simulink model "lab_modulation_am"  (R2022a)
settings: Solver=VariableStepAuto  StartTime=0.0  StopTime=10.0  RelTol=1e-3
libraries: dspfdesign x1
settings Model: Creator=salgi  LastModifiedBy=salgi

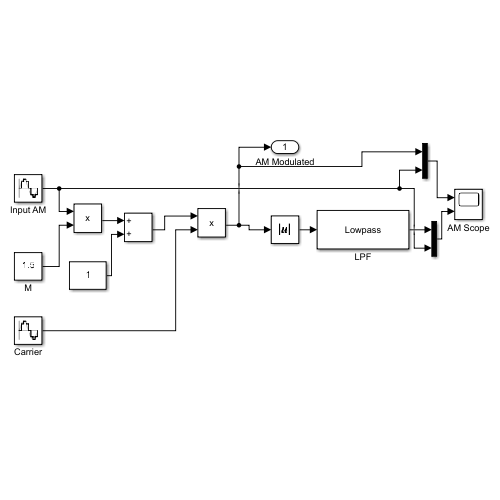
[thumbnail: Simulink's stored preview of the top-level diagram]
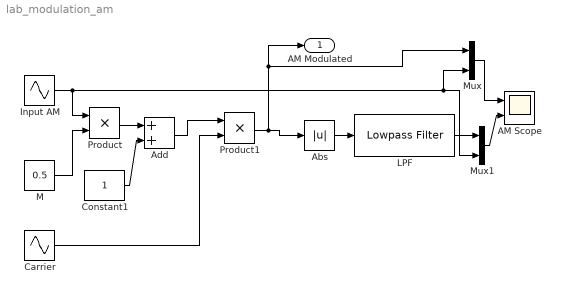
== system lab_modulation_am ==
  AM Scope : Scope  NumInputPorts=2
  Abs : Abs  SaturateOnIntegerOverflow=off
  Add : Sum
  Carrier : Sin  Frequency=100*2*pi  SampleTime=0.0001
  Constant1 : Constant
  Input AM : Sin  Frequency=2*2*pi  SampleTime=0.0001
  LPF : dspfdesign/Lowpass Filter  FilterType=FIR  DesignForMinimumOrder=on  FilterOrder=50  PassbandFrequency=0.1  StopbandFrequency=100  PassbandRipple=0.1  StopbandAttenuation=80  InheritSampleRate=on  SampleRate=44100  SimulateUsing=Interpreted execution  roundingMode=Floor  coeffsDataTypeStr=fixdt(1,16)
  M : Constant  Value=0.5
  Mux : Mux  Inputs=2
  Mux1 : Mux  Inputs=2
  Product : Product
  Product1 : Product
  AM Modulated : Outport
  wires:
  Mux/1 -> AM Scope/1
  Input AM/1 -> Mux/2, Mux1/2, Product/1
  Carrier/1 -> Product1/2
  Product1/1 -> Mux/1, AM Modulated/1, Abs/1
  Abs/1 -> LPF/1
  Constant1/1 -> Add/2
  M/1 -> Product/2
  Mux1/1 -> AM Scope/2
  Product/1 -> Add/1
  Add/1 -> Product1/1
  LPF/1 -> Mux1/1
